simulink subsystem "GridConnectInverter"  (R2020a)
settings: Solver=VariableStepAuto  StartTime=0.0  StopTime=10.0  RelTol=1e-3
libraries: ee_lib x12, nesl_utility x6, eePwmGenerator x4, fl_lib x2
settings Model: Creator=ykamatan  LastModifiedBy=ykamatan

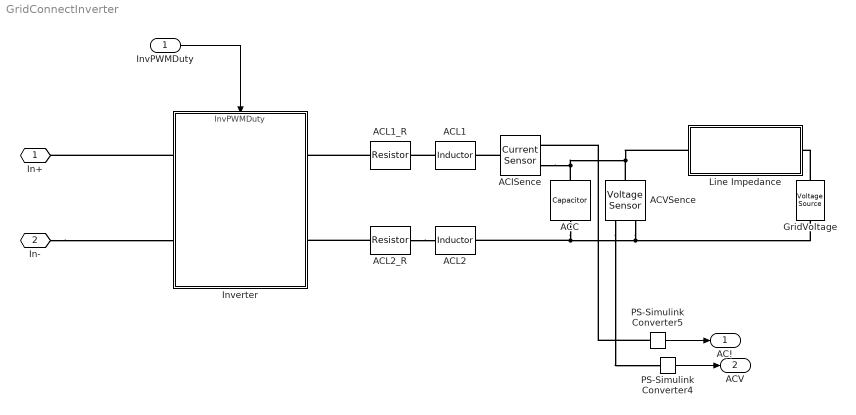
== system GridConnectInverter ==
  InvPWMDuty : Inport
  ACC : ee_lib/Passive/Capacitor  cap_option=0  c=1e-6 F  Cvec=[1e-05, 1e-06] F  Vvec=[0, 10] V  CV_table_symmetry=1  f_vec=[1, 10] kHz  DFext_vec=[.8, 1.2]  C_tol=5  enable_C_tol=0  tol_distribution=1  nSigma=4  r=1e-6 Ohm  g=0 1/Ohm  averaging_period=0 s  enable_operating_limits=0  operating_limit_action=2  max_working_voltage_range=[-25, 25] V  power_rating=1 W  enable_faults=0  fault_action=1  Cscale_faulted=100  R_faulted=1e-3 Ohm  G_faulted=0 1/Ohm  tau_fault=1e-3 s  enable_temporal_fault=0  t_fault=1 s  enable_behavioral_fault=0  max_permissible_voltage_range=[-100, 100] V  t_fail_on_voltage=1 s  i_specify=off  i_priority=None  i=0 A  i_nominal_specify=off  i_nominal_unit=A  i_nominal_value=1  v_specify=off  v_priority=None  v=0 V  v_nominal_specify=off  v_nominal_unit=V  v_nominal_value=1  vc_specify=off  vc_priority=High  vc=0 V  vc_nominal_specify=off  vc_nominal_unit=V  vc_nominal_value=1
  ACISence : fl_lib/Electrical/Electrical Sensors/Current Sensor
  ACL1 : ee_lib/Passive/Inductor  l=1e-6 H  L_tol=20  enable_L_tol=0  tol_distribution=1  nSigma=4  r=0 Ohm  g=1e-9 1/Ohm  enable_operating_limits=0  operating_limit_action=2  max_working_current=1 A  power_rating=1 W  enable_faults=0  fault_action=1  lambdaPercent=50  k_faulted=0.9999  turnsShort=0  openCct=0  groundShort=0  groundShortG=0 1/Ohm  tau_fault=1e-3 s  enable_temporal_fault=0  t_fault=1 s  enable_behavioral_fault=0  max_permissible_voltage=100 V  n_fail_on_voltage=1  max_permissible_current=1 A  t_fail_on_current=1 s  i_L_specify=off  i_L_priority=High  i_L=0 A  i_L_nominal_specify=off  i_L_nominal_unit=A  i_L_nominal_value=1
  ACL1_R : ee_lib/Passive/Resistor  R=1 Ohm  R_tol=5  enable_R_tol=0  tol_distribution=1  nSigma=4  enable_operating_limits=0  operating_limit_action=2  max_working_voltage=100 V  power_rating=1 W  enable_faults=0  fault_action=1  R_faulted=inf Ohm  enable_temporal_fault=0  t_fault=1 s  enable_behavioral_fault=0  max_permissible_current=1 A  t_fail_on_current=1 s  noise_mode=0  sample_time=1e-3 s  repeatability=1  auto_seed=2061249901  user_seed=0  Tdevice=25 degC  alpha=3.93e-3 1/K  Tmeas=25 degC  thermal_mass=100 J/K  power_derating_T1=70 degC  power_derating_T2=155 degC  operating_temperature_range_vec=[-50, 150] degC  temperature_specify=off  temperature_priority=High  temperature=298.15 K  temperature_nominal_specify=off  temperature_nominal_unit=K  temperature_nominal_value=1
  ACL2 : ee_lib/Passive/Inductor  l=1e-6 H  L_tol=20  enable_L_tol=0  tol_distribution=1  nSigma=4  r=0 Ohm  g=1e-9 1/Ohm  enable_operating_limits=0  operating_limit_action=2  max_working_current=1 A  power_rating=1 W  enable_faults=0  fault_action=1  lambdaPercent=50  k_faulted=0.9999  turnsShort=0  openCct=0  groundShort=0  groundShortG=0 1/Ohm  tau_fault=1e-3 s  enable_temporal_fault=0  t_fault=1 s  enable_behavioral_fault=0  max_permissible_voltage=100 V  n_fail_on_voltage=1  max_permissible_current=1 A  t_fail_on_current=1 s  i_L_specify=off  i_L_priority=High  i_L=0 A  i_L_nominal_specify=off  i_L_nominal_unit=A  i_L_nominal_value=1
  ACL2_R : ee_lib/Passive/Resistor  R=1 Ohm  R_tol=5  enable_R_tol=0  tol_distribution=1  nSigma=4  enable_operating_limits=0  operating_limit_action=2  max_working_voltage=100 V  power_rating=1 W  enable_faults=0  fault_action=1  R_faulted=inf Ohm  enable_temporal_fault=0  t_fault=1 s  enable_behavioral_fault=0  max_permissible_current=1 A  t_fail_on_current=1 s  noise_mode=0  sample_time=1e-3 s  repeatability=1  auto_seed=3885752424  user_seed=0  Tdevice=25 degC  alpha=3.93e-3 1/K  Tmeas=25 degC  thermal_mass=100 J/K  power_derating_T1=70 degC  power_derating_T2=155 degC  operating_temperature_range_vec=[-50, 150] degC  temperature_specify=off  temperature_priority=High  temperature=298.15 K  temperature_nominal_specify=off  temperature_nominal_unit=K  temperature_nominal_value=1
  ACVSence : fl_lib/Electrical/Electrical Sensors/Voltage Sensor
  GridVoltage : ee_lib/Sources/Voltage Source  dc_voltage=0 V  ac_voltage=202 V  ac_shift=0 rad  ac_frequency=60 Hz  noise_mode=0  PSD=0 V^2/Hz  repeatability=1  auto_seed=2619357310  user_seed=0  sample_time=1e-3 s  i_specify=off  i_priority=None  i=0 A  i_nominal_specify=off  i_nominal_unit=A  i_nominal_value=1  v_specify=off  v_priority=None  v=0 V  v_nominal_specify=off  v_nominal_unit=V  v_nominal_value=1
  Inverter : Subsystem
      settings: PortSchema="{\"entries\":[{\"content\":{\"sides\":[{\"content\":{\"connectorIds\":[\"LConn1\",\"LConn2\"]},\"type\":\"ConnectorPlacement.EquallySpacedRectSide\",\"uuid\":\"5516e6e0-e90b-45b6-9097-7d81db5529b7\"},{\"content\":{\"connectorIds\":[\"RConn1\",\"RConn2\"],\"side\":\"RIGHT\"},\"type\":\"ConnectorPlacement.EquallySpacedRectSide\",\"uuid\":\"c08daa1d-3c8d-4022-a135-6251002e3faa\"},{\"content\":{\"connectorIds\":[\"In1\"],\"side\":\"TOP\"},\"type\":\"ConnectorPlacement.EquallySpacedRectSide\",\"uuid\":\"063f088e-77c7-44ca-915a-d9d0d7c33669\"}]},\"type\":\"ConnectorPlacement.EquallySpacedConnector\",\"uuid\":\"98f901b5-3d53-45dd-ae63-ab694af0ed2d\"}],\"packageUris\":[\"http://schema.mathworks.com/mf0/Connector/19700101\"],\"version\":\"1.0\"}"
  Line Impedance : Subsystem
  PS-Simulink Converter4 : nesl_utility/PS-Simulink Converter  PhysicalDomain=network_engine_domain  SubClassName=ps_output  LeftPortType=input  RightPortType=output  PseudoPeriodic=off  Frequencies=[]  Unit=inherit  AffineConversion=off
  PS-Simulink Converter5 : nesl_utility/PS-Simulink Converter  PhysicalDomain=network_engine_domain  SubClassName=ps_output  LeftPortType=input  RightPortType=output  PseudoPeriodic=off  Frequencies=[]  Unit=inherit  AffineConversion=off
  In+ : PMIOPort  Side=Left
  In- : PMIOPort  Port=2  Side=Left
  AC! : Outport
  ACV : Outport  Port=2
  wires:
  InvPWMDuty/1 -> Inverter/1(InvPWMDuty)
  PS-Simulink Converter5/1 -> AC!/1
  PS-Simulink Converter4/1 -> ACV/1
  connections:
  ACC/RConn1 -- ACL2/LConn1 -- GridVoltage/RConn1 -- ACVSence/RConn2
  ACISence/RConn2 -- ACC/LConn1 -- ACVSence/LConn1 -- Line Impedance/LConn1
  ACISence/LConn1 -- ACL1/RConn1
  ACL1_R/LConn1 -- Inverter/RConn1
  ACL2_R/LConn1 -- ACL2/RConn1
  GridVoltage/LConn1 -- Line Impedance/RConn1
  In-/RConn1 -- Inverter/LConn2
  ACL1/LConn1 -- ACL1_R/RConn1
  ACL2_R/RConn1 -- Inverter/RConn2
  PS-Simulink Converter5/LConn1 -- ACISence/RConn1
  ACVSence/RConn1 -- PS-Simulink Converter4/LConn1
  Inverter/LConn1 -- In+/RConn1

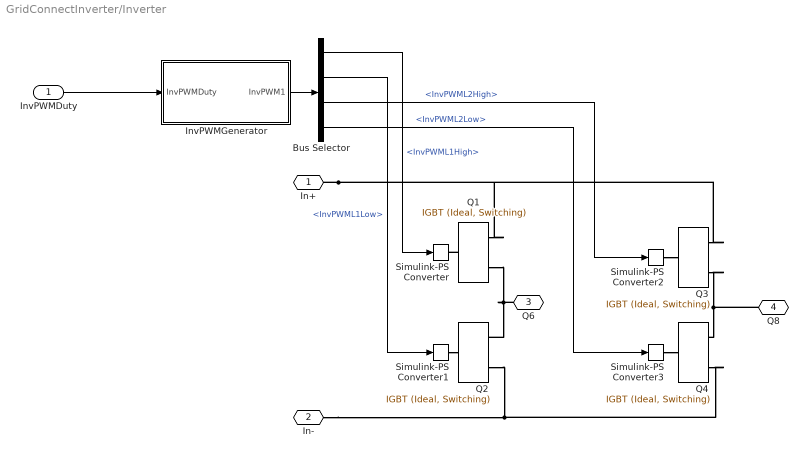
== system GridConnectInverter/Inverter ==
  InvPWMDuty : Inport
  Bus Selector : BusSelector  OutputSignals=InvPWML1High,InvPWML1Low,InvPWML2High,InvPWML2Low
  InvPWMGenerator : Subsystem
  Q{1..4} (4 alike) : ee_lib/Semiconductors & Converters/IGBT (Ideal, Switching)  Vf=0.8 V  Ron=0.001 Ohm  Goff=1e-5 1/Ohm  Vth=6 V  diode_param=1  diode_Vf=0.8 V  diode_Ron=0.001 Ohm  diode_Goff=1e-5 1/Ohm  diode_C=50e-9 F  diode_iRM=-235 A  diode_iF=300 A  diode_idot=-50 A/us  diode_trr_param=1  diode_trr_factor=3  diode_trr=15 us  diode_Qrr=1500 s*uA  thermal_loss_option=2  Voff=300 V  Tau=1e-4 s  Tj=[298.15, 398.15] K  Iout_scalar=600 A  Eon_scalar=22.86e-3 J  Eoff_scalar=17.14e-3 J  Von_scalar=2.7 V  Iout_data=[0, 10, 50, 100, 200, 400, 600] A  Eon_data=[0, .29, 1.43, 2.86, 5.71, 13.14, 22.86; 0, .57, 2.63, 5.14, 10.29, 20.57, 30.29] * 1e-3 J  Eoff_data=[0, .21, 1.07, 2.14, 4.29, 9.86, 17.14; 0, .43, 1.97, 3.86, 7.71, 15.43, 22.71] * 1e-3 J  Von_data=[0, 1.1, 1.3, 1.45, 1.75, 2.25, 2.7; 0, 1, 1.15, 1.35, 1.7, 2.35, 3] V
  Simulink-PS Converter{,1..3} (4 alike) : nesl_utility/Simulink-PS Converter  PhysicalDomain=network_engine_domain  SubClassName=ps_input  LeftPortType=input  RightPortType=output  PseudoPeriodic=off  Frequencies=[]  NoiseDistribution=none  NoiseParameters=[]  Unit=1  AffineConversion=off  FilteringAndDerivatives=provide  SimscapeFilterOrder=1  InputFilterTimeConstant=0.001  UdotUserProvided=0
  In+ : PMIOPort  Side=Left
  In- : PMIOPort  Port=2  Side=Left
  Q6 : PMIOPort  Port=3  Side=Right
  Q8 : PMIOPort  Port=4  Side=Right
  wires:
  InvPWMDuty/1 -> InvPWMGenerator/1(InvPWMDuty)
  Bus Selector/1 -> Simulink-PS Converter/1  "<InvPWML1High>"
  Bus Selector/3 -> Simulink-PS Converter2/1  "<InvPWML2High>"
  Bus Selector/4 -> Simulink-PS Converter3/1  "<InvPWML2Low>"
  Bus Selector/2 -> Simulink-PS Converter1/1  "<InvPWML1Low>"
  InvPWMGenerator/1(InvPWM1) -> Bus Selector/1
  connections:
  Q1/LConn1 -- Simulink-PS Converter/RConn1
  In+/RConn1 -- Q1/RConn1 -- Q3/RConn1
  Simulink-PS Converter2/RConn1 -- Q3/LConn1
  Simulink-PS Converter3/RConn1 -- Q4/LConn1
  In-/RConn1 -- Q2/RConn2 -- Q4/RConn2
  Simulink-PS Converter1/RConn1 -- Q2/LConn1
  Q8/RConn1 -- Q4/RConn1 -- Q3/RConn2
  Q6/RConn1 -- Q2/RConn1 -- Q1/RConn2

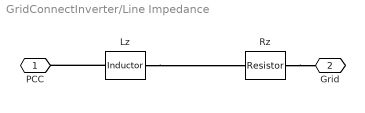
== system GridConnectInverter/Line Impedance ==
  Lz : ee_lib/Passive/Inductor  l=1e-6 H  L_tol=20  enable_L_tol=0  tol_distribution=1  nSigma=4  r=0 Ohm  g=1e-9 1/Ohm  enable_operating_limits=0  operating_limit_action=2  max_working_current=1 A  power_rating=1 W  enable_faults=0  fault_action=1  lambdaPercent=50  k_faulted=0.9999  turnsShort=0  openCct=0  groundShort=0  groundShortG=0 1/Ohm  tau_fault=1e-3 s  enable_temporal_fault=0  t_fault=1 s  enable_behavioral_fault=0  max_permissible_voltage=100 V  n_fail_on_voltage=1  max_permissible_current=1 A  t_fail_on_current=1 s  i_L_specify=off  i_L_priority=High  i_L=0 A  i_L_nominal_specify=off  i_L_nominal_unit=A  i_L_nominal_value=1
  Rz : ee_lib/Passive/Resistor  R=1 Ohm  R_tol=5  enable_R_tol=0  tol_distribution=1  nSigma=4  enable_operating_limits=0  operating_limit_action=2  max_working_voltage=100 V  power_rating=1 W  enable_faults=0  fault_action=1  R_faulted=inf Ohm  enable_temporal_fault=0  t_fault=1 s  enable_behavioral_fault=0  max_permissible_current=1 A  t_fail_on_current=1 s  noise_mode=0  sample_time=1e-3 s  repeatability=1  auto_seed=2652856943  user_seed=0  Tdevice=25 degC  alpha=3.93e-3 1/K  Tmeas=25 degC  thermal_mass=100 J/K  power_derating_T1=70 degC  power_derating_T2=155 degC  operating_temperature_range_vec=[-50, 150] degC  temperature_specify=off  temperature_priority=High  temperature=298.15 K  temperature_nominal_specify=off  temperature_nominal_unit=K  temperature_nominal_value=1
  PCC : PMIOPort  Side=Left
  Grid : PMIOPort  Port=2  Side=Right
  connections:
  Rz/RConn1 -- Grid/RConn1
  Lz/RConn1 -- Rz/LConn1
  Lz/LConn1 -- PCC/RConn1

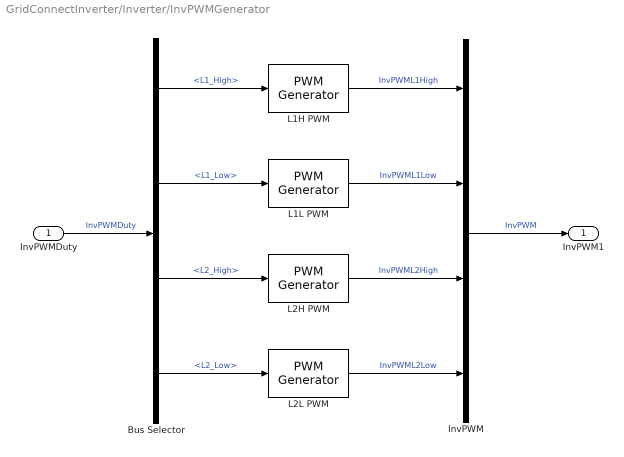
== system GridConnectInverter/Inverter/InvPWMGenerator ==
  InvPWMDuty : Inport
  Bus Selector : BusSelector  OutputSignals=L1_High,L1_Low,L2_High,L2_Low
  InvPWM : BusCreator  Inputs=4
  L1H PWM : eePwmGenerator/PWM Generator  CarrCount=Up  Tper=0.001  Ts=5e-5
  L1L PWM : eePwmGenerator/PWM Generator  CarrCount=Up  Tper=0.001  Ts=5e-5
  L2H PWM : eePwmGenerator/PWM Generator  CarrCount=Up  Tper=0.001  Ts=5e-5
  L2L PWM : eePwmGenerator/PWM Generator  CarrCount=Up  Tper=0.001  Ts=5e-5
  InvPWM1 : Outport
  wires:
  InvPWM/1 -> InvPWM1/1  "InvPWM"
  Bus Selector/4 -> L2L PWM/1  "<L2_Low>"
  L1H PWM/1 -> InvPWM/1  "InvPWML1High"
  L1L PWM/1 -> InvPWM/2  "InvPWML1Low"
  Bus Selector/1 -> L1H PWM/1  "<L1_High>"
  L2H PWM/1 -> InvPWM/3  "InvPWML2High"
  Bus Selector/3 -> L2H PWM/1  "<L2_High>"
  L2L PWM/1 -> InvPWM/4  "InvPWML2Low"
  InvPWMDuty/1 -> Bus Selector/1  "InvPWMDuty"
  Bus Selector/2 -> L1L PWM/1  "<L1_Low>"
